simulink model "CL_MI_ARMAX"  (R2015a)
settings: Solver=ode45  StartTime=0.0  StopTime=520  RelTol=1e-3
values from neighbouring files (symbols this model uses):
  lambda = 1    [generar_prbs.m]    (also in parametros_ident.m = 0.995)
  Ts = 0.01    [generar_prbs.m]
libraries: dspsigops x2
settings Model: Creator=u_labelectro  LastModifiedBy=ARTURO
settings DataIOCC: SignalLoggingSaveFormat=ModelDataLogs
settings DebuggingCC: UnderspecifiedInitializationDetection=Classic  MergeDetectMultiDrivingBlocksExec=none  SolverPrmCheckMsg=warning  MultiTaskDSMMsg=warning  MultiTaskCondExecSysMsg=none  StateNameClashWarn=warning

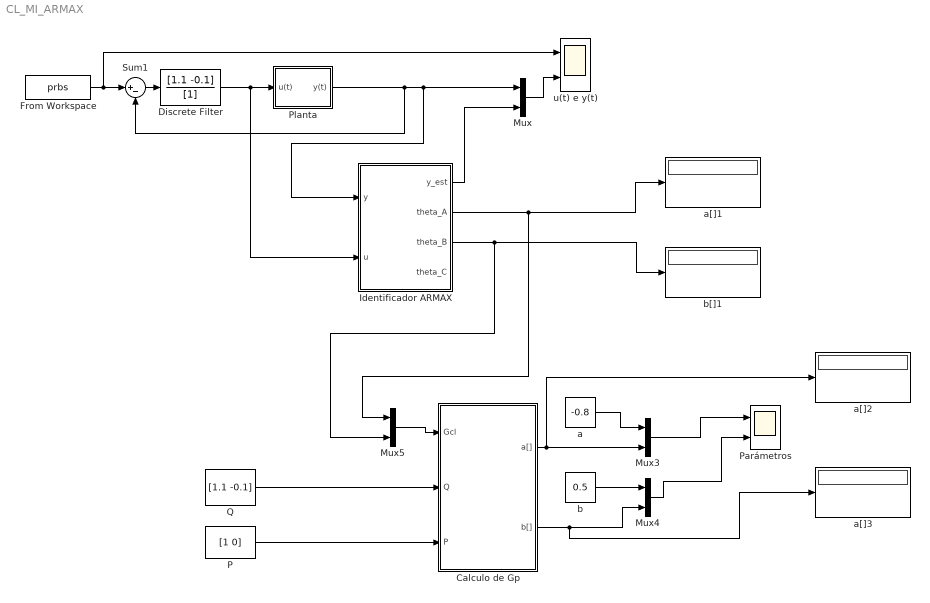
== system CL_MI_ARMAX ==
  Calculo de Gp : Subsystem
  Discrete Filter : DiscreteFilter  Numerator=[1.1 -0.1]  Denominator=[1]
  From Workspace : FromWorkspace  VariableName=prbs  SampleTime=Ts
  Identificador ARMAX : Subsystem
  Mux{,3..5} (4 alike) : Mux  Inputs=2
  P : Constant  Value=[1 0]
  Parámetros : Scope  NumInputPorts=2
      settings: YMin=-5~-5  YMax=5~5  SaveName=ScopeData4
  Planta : Subsystem
  Q : Constant  Value=[1.1 -0.1]
  Sum1 : Sum  Inputs=|+-
  a : Constant  Value=-0.8
  a[]1 : Display
  a[]2 : Display
  a[]3 : Display
  b : Constant  Value=0.5
  b[]1 : Display
  u(t) e y(t) : Scope  NumInputPorts=2
      settings: YMin=-5~-5  YMax=5~5
  wires:
  Identificador ARMAX/1(y_est) -> Mux/2
  Identificador ARMAX/3(theta_B) -> Mux5/2, b[]1/1
  Mux/1 -> u(t) e y(t)/2
  Discrete Filter/1 -> Identificador ARMAX/2(u), Planta/1(u(t))
  From Workspace/1 -> Sum1/1, u(t) e y(t)/1
  Planta/1(y(t)) -> Sum1/2, Identificador ARMAX/1(y), Mux/1
  a/1 -> Mux3/1
  b/1 -> Mux4/1
  Mux3/1 -> Parámetros/1
  Mux4/1 -> Parámetros/2
  Calculo de Gp/2(b[]) -> a[]3/1, Mux4/2
  Mux5/1 -> Calculo de Gp/1(Gcl)
  Q/1 -> Calculo de Gp/2(Q)
  P/1 -> Calculo de Gp/3(P)
  Identificador ARMAX/2(theta_A) -> Mux5/1, a[]1/1
  Calculo de Gp/1(a[]) -> a[]2/1, Mux3/2
  Sum1/1 -> Discrete Filter/1

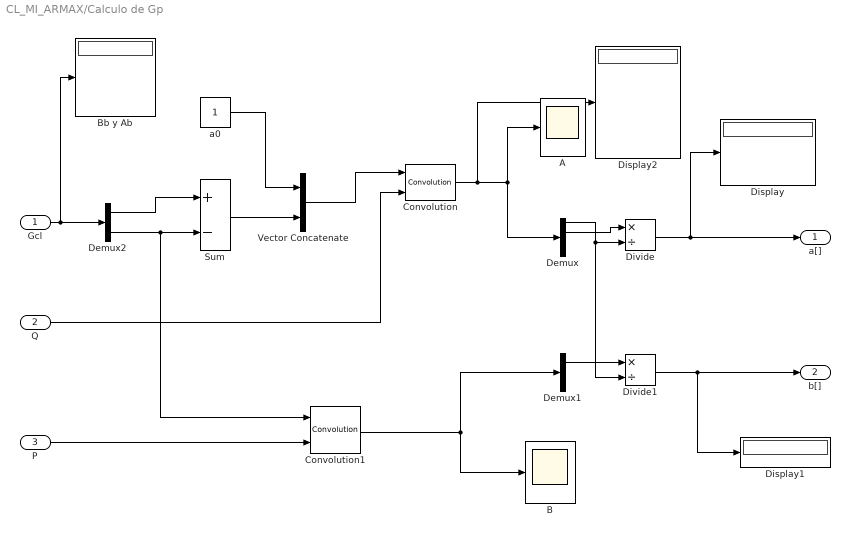
== system CL_MI_ARMAX/Calculo de Gp ==
  Gcl : Inport
  Q : Inport  Port=2
  P : Inport  Port=3
  A : Scope
      settings: SaveName=ScopeData2
  B : Scope
      settings: SaveName=ScopeData3
  "Bb y Ab " : Display
  Convolution : dspsigops/Convolution  domain=Time  outputDataTypeStr=Inherit: Same as accumulator  outputLastDataTypeStr=Inherit: Same as accumulator  outputMin=[]  outputMax=[]  roundingMode=Floor  overflowMode=off
  Convolution1 : dspsigops/Convolution  domain=Time  outputDataTypeStr=Inherit: Same as accumulator  outputLastDataTypeStr=Inherit: Same as accumulator  outputMin=[]  outputMax=[]  roundingMode=Floor  overflowMode=off
  Demux : Demux
  Demux1 : Demux  Outputs=3
  Demux2 : Demux  Outputs=2
  Display : Display
  Display1 : Display
  Display2 : Display
  Divide : Product  Inputs=*/
  Divide1 : Product  Inputs=*/
  Sum : Sum  Inputs=+-
  Vector Concatenate : Concatenate
  a0 : Constant
  a[] : Outport
  b[] : Outport  Port=2
  wires:
  Gcl/1 -> "Bb y Ab "/1, Demux2/1
  Demux2/2 -> Convolution1/1, Sum/2
  Demux2/1 -> Sum/1
  a0/1 -> Vector Concatenate/1
  Sum/1 -> Vector Concatenate/2
  Divide1/1 -> Display1/1, b[]/1
  Divide/1 -> Display/1, a[]/1
  Demux1/1 -> Divide1/1
  Demux/1 -> Divide/2, Divide1/2
  Demux/2 -> Divide/1
  Convolution1/1 -> Demux1/1, B/1
  Convolution/1 -> Display2/1, A/1, Demux/1
  Vector Concatenate/1 -> Convolution/1
  Q/1 -> Convolution/2
  P/1 -> Convolution1/2

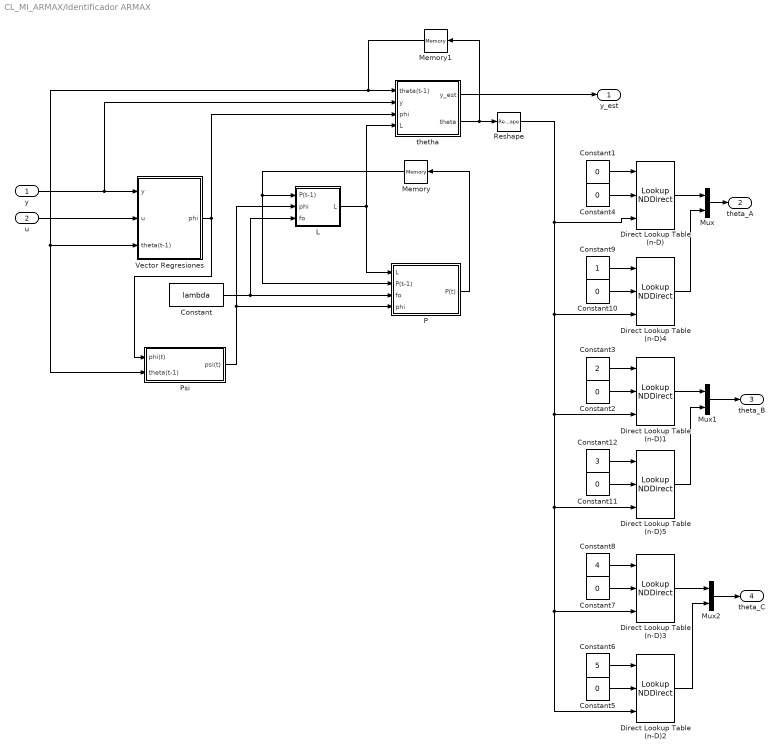
== system CL_MI_ARMAX/Identificador ARMAX ==
  y : Inport
  u : Inport  Port=2
  Constant : Constant  Value=lambda
  Constant{1..2,4..5,7,10..11} (7 alike) : Constant  Value=0
  Constant12 : Constant  Value=3
  Constant3 : Constant  Value=2
  Constant6 : Constant  Value=5
  Constant8 : Constant  Value=4
  Constant9 : Constant
  Direct Lookup Table (n-D){,1..5} (6 alike) : LookupNDDirect  TableIsInput=on
  L : Subsystem
  Memory : Memory  X0=1e6*eye(6)
  Memory1 : Memory
  Mux : Mux  Inputs=2
  Mux1 : Mux  Inputs=2
  Mux2 : Mux  Inputs=2
  P : Subsystem
  Psi : Subsystem
  Reshape : Reshape  OutputDimensionality=Column vector (2-D)
  Vector Regresiones : Subsystem
  thetha : Subsystem
  y_est : Outport
  theta_A : Outport  Port=2
  theta_B : Outport  Port=3
  theta_C : Outport  Port=4
  wires:
  y/1 -> thetha/2(y), Vector Regresiones/1(y)
  u/1 -> Vector Regresiones/2(u)
  L/1(L) -> thetha/4(L), P/1(L)
  P/1(P(t)) -> Memory/1
  Memory/1 -> P/2(P(t-1)), L/1(P(t-1))
  thetha/2(theta) -> Memory1/1, Reshape/1
  Memory1/1 -> Vector Regresiones/3(theta(t-1)), Psi/2(theta(t-1)), thetha/1(theta(t-1))
  thetha/1(y_est) -> y_est/1
  Constant1/1 -> Direct Lookup Table (n-D)/1
  Constant4/1 -> Direct Lookup Table (n-D)/2
  Constant3/1 -> Direct Lookup Table (n-D)1/1
  Constant2/1 -> Direct Lookup Table (n-D)1/2
  Constant/1 -> L/3(fo), P/3(fo)
  Psi/1(psi(t)) -> L/2(phi), P/4(phi)
  Vector Regresiones/1(phi) -> Psi/1(phi(t)), thetha/3(phi)
  Constant5/1 -> Direct Lookup Table (n-D)2/2
  Constant6/1 -> Direct Lookup Table (n-D)2/1
  Constant7/1 -> Direct Lookup Table (n-D)3/2
  Constant8/1 -> Direct Lookup Table (n-D)3/1
  Constant9/1 -> Direct Lookup Table (n-D)4/1
  Constant10/1 -> Direct Lookup Table (n-D)4/2
  Constant12/1 -> Direct Lookup Table (n-D)5/1
  Constant11/1 -> Direct Lookup Table (n-D)5/2
  Reshape/1 -> Direct Lookup Table (n-D)5/3, Direct Lookup Table (n-D)2/3, Direct Lookup Table (n-D)3/3, Direct Lookup Table (n-D)1/3, Direct Lookup Table (n-D)4/3, Direct Lookup Table (n-D)/3
  Direct Lookup Table (n-D)/1 -> Mux/1
  Mux/1 -> theta_A/1
  Direct Lookup Table (n-D)4/1 -> Mux/2
  Mux2/1 -> theta_C/1
  Mux1/1 -> theta_B/1
  Direct Lookup Table (n-D)1/1 -> Mux1/1
  Direct Lookup Table (n-D)5/1 -> Mux1/2
  Direct Lookup Table (n-D)3/1 -> Mux2/1
  Direct Lookup Table (n-D)2/1 -> Mux2/2

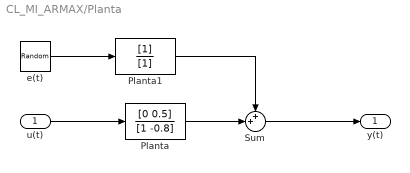
== system CL_MI_ARMAX/Planta ==
  u(t) : Inport
  Planta : DiscreteFilter  Numerator=[0 0.5]  Denominator=[1 -0.8]  SampleTime=Ts
  Planta1 : DiscreteFilter  Denominator=[1]  SampleTime=Ts
  Sum : Sum  Inputs=++|
  e(t) : RandomNumber  Variance=0.0001  SampleTime=Ts
  y(t) : Outport
  wires:
  e(t)/1 -> Planta1/1
  Planta1/1 -> Sum/1
  Planta/1 -> Sum/2
  u(t)/1 -> Planta/1
  Sum/1 -> y(t)/1

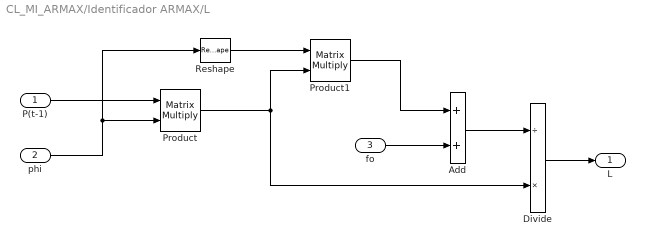
== system CL_MI_ARMAX/Identificador ARMAX/L ==
  P(t-1) : Inport
  phi : Inport  Port=2
  fo : Inport  Port=3
  Add : Sum
  Divide : Product  Inputs=/*
  Product : Product  Multiplication=Matrix(*)
  Product1 : Product  Multiplication=Matrix(*)
  Reshape : Reshape  OutputDimensionality=Row vector (2-D)
  L : Outport
  wires:
  phi/1 -> Reshape/1, Product/2
  P(t-1)/1 -> Product/1
  Reshape/1 -> Product1/1
  fo/1 -> Add/2
  Product1/1 -> Add/1
  Divide/1 -> L/1
  Add/1 -> Divide/1
  Product/1 -> Divide/2, Product1/2

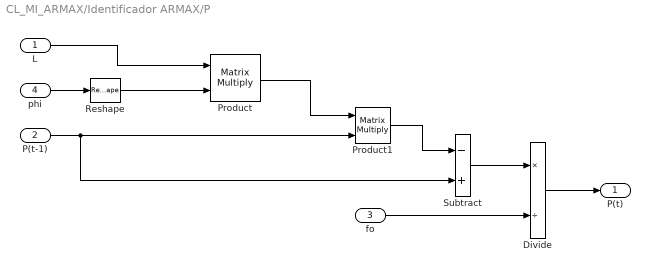
== system CL_MI_ARMAX/Identificador ARMAX/P ==
  L : Inport
  P(t-1) : Inport  Port=2
  fo : Inport  Port=3
  phi : Inport  Port=4
  Divide : Product  Inputs=*/
  Product : Product  Multiplication=Matrix(*)
  Product1 : Product  Multiplication=Matrix(*)
  Reshape : Reshape  OutputDimensionality=Row vector (2-D)
  Subtract : Sum  Inputs=-+
  P(t) : Outport
  wires:
  phi/1 -> Reshape/1
  Reshape/1 -> Product/2
  L/1 -> Product/1
  Product/1 -> Product1/1
  P(t-1)/1 -> Subtract/2, Product1/2
  Product1/1 -> Subtract/1
  Subtract/1 -> Divide/1
  fo/1 -> Divide/2
  Divide/1 -> P(t)/1

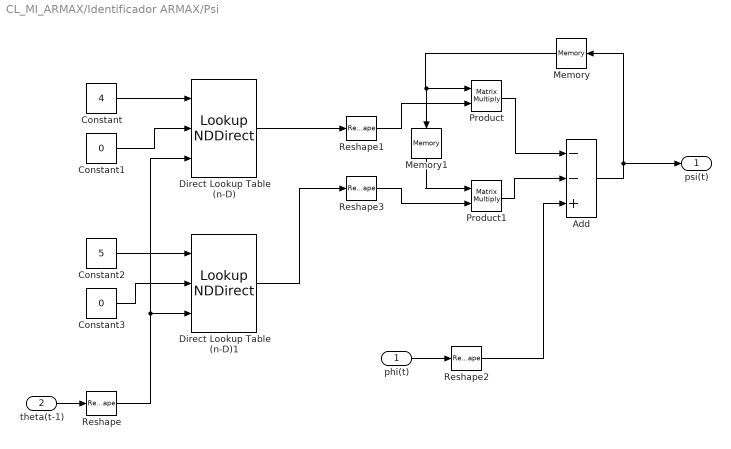
== system CL_MI_ARMAX/Identificador ARMAX/Psi ==
  phi(t) : Inport
  theta(t-1) : Inport  Port=2
  Add : Sum  Inputs=--+
  Constant : Constant  Value=4
  Constant1 : Constant  Value=0
  Constant2 : Constant  Value=5
  Constant3 : Constant  Value=0
  Direct Lookup Table (n-D) : LookupNDDirect  TableIsInput=on
  Direct Lookup Table (n-D)1 : LookupNDDirect  TableIsInput=on
  Memory : Memory
  Memory1 : Memory
  Product : Product  Multiplication=Matrix(*)
  Product1 : Product  Multiplication=Matrix(*)
  Reshape : Reshape  OutputDimensionality=Column vector (2-D)
  Reshape1 : Reshape  OutputDimensionality=Row vector (2-D)
  Reshape2 : Reshape  OutputDimensionality=Column vector (2-D)
  Reshape3 : Reshape  OutputDimensionality=Row vector (2-D)
  psi(t) : Outport
  wires:
  Constant/1 -> Direct Lookup Table (n-D)/1
  Constant1/1 -> Direct Lookup Table (n-D)/2
  theta(t-1)/1 -> Reshape/1
  Reshape/1 -> Direct Lookup Table (n-D)1/3, Direct Lookup Table (n-D)/3
  Reshape1/1 -> Product/2
  Product/1 -> Add/1
  phi(t)/1 -> Reshape2/1
  Add/1 -> Memory/1, psi(t)/1
  Constant2/1 -> Direct Lookup Table (n-D)1/1
  Constant3/1 -> Direct Lookup Table (n-D)1/2
  Direct Lookup Table (n-D)1/1 -> Reshape3/1
  Direct Lookup Table (n-D)/1 -> Reshape1/1
  Memory/1 -> Memory1/1, Product/1
  Reshape2/1 -> Add/3
  Product1/1 -> Add/2
  Reshape3/1 -> Product1/2
  Memory1/1 -> Product1/1

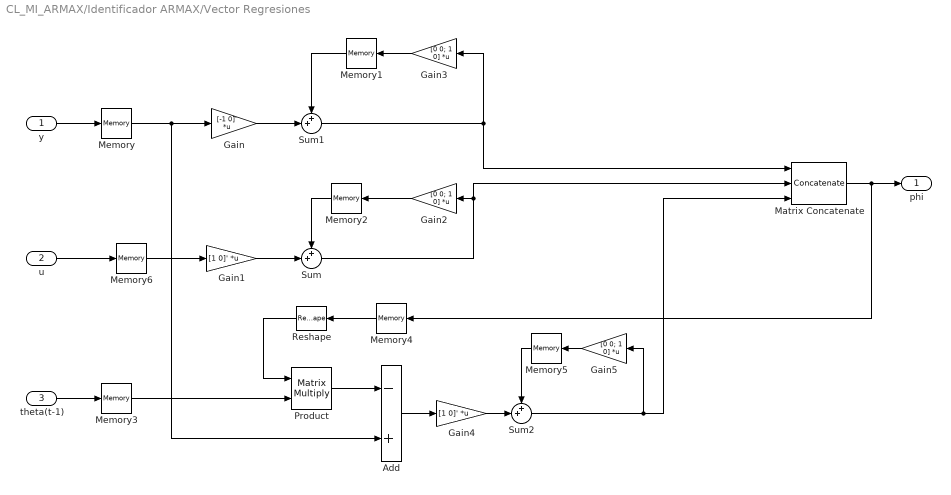
== system CL_MI_ARMAX/Identificador ARMAX/Vector Regresiones ==
  y : Inport
  u : Inport  Port=2
  theta(t-1) : Inport  Port=3
  Add : Sum  Inputs=-+
  Gain : Gain  Gain=[-1 0]'  Multiplication=Matrix(K*u)
  Gain1 : Gain  Gain=[1 0]'  Multiplication=Matrix(K*u)
  Gain2 : Gain  Gain=[0 0; 1 0]  Multiplication=Matrix(K*u)
  Gain3 : Gain  Gain=[0 0; 1 0]  Multiplication=Matrix(K*u)
  Gain4 : Gain  Gain=[1 0]'  Multiplication=Matrix(K*u)
  Gain5 : Gain  Gain=[0 0; 1 0]  Multiplication=Matrix(K*u)
  Matrix Concatenate : Concatenate  NumInputs=3  Mode=Multidimensional array
  Memory{,1..6} (7 alike) : Memory
  Product : Product  Multiplication=Matrix(*)
  Reshape : Reshape  OutputDimensionality=Row vector (2-D)
  Sum : Sum  Inputs=++|
  Sum1 : Sum  Inputs=++|
  Sum2 : Sum  Inputs=++|
  phi : Outport
  wires:
  y/1 -> Memory/1
  Memory2/1 -> Sum/1
  Gain1/1 -> Sum/2
  Gain2/1 -> Memory2/1
  Memory1/1 -> Sum1/1
  Gain3/1 -> Memory1/1
  Memory/1 -> Add/2, Gain/1
  Matrix Concatenate/1 -> Memory4/1, phi/1
  Sum1/1 -> Matrix Concatenate/1, Gain3/1
  Sum/1 -> Matrix Concatenate/2, Gain2/1
  theta(t-1)/1 -> Memory3/1
  Memory3/1 -> Product/2
  Reshape/1 -> Product/1
  Memory4/1 -> Reshape/1
  Product/1 -> Add/1
  Add/1 -> Gain4/1
  Gain4/1 -> Sum2/2
  Gain5/1 -> Memory5/1
  Memory5/1 -> Sum2/1
  Sum2/1 -> Gain5/1, Matrix Concatenate/3
  Gain/1 -> Sum1/2
  u/1 -> Memory6/1
  Memory6/1 -> Gain1/1

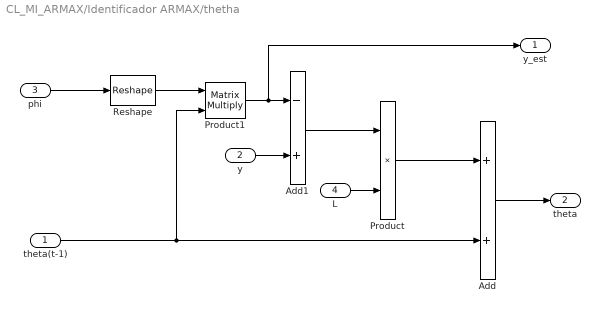
== system CL_MI_ARMAX/Identificador ARMAX/thetha ==
  theta(t-1) : Inport
  y : Inport  Port=2
  phi : Inport  Port=3
  L : Inport  Port=4
  Add : Sum
  Add1 : Sum  Inputs=-+
  Product : Product
  Product1 : Product  Multiplication=Matrix(*)
  Reshape : Reshape  OutputDimensionality=Row vector (2-D)
  y_est : Outport
  theta : Outport  Port=2
  wires:
  phi/1 -> Reshape/1
  y/1 -> Add1/2
  L/1 -> Product/2
  Add1/1 -> Product/1
  Product/1 -> Add/1
  theta(t-1)/1 -> Add/2, Product1/2
  Reshape/1 -> Product1/1
  Product1/1 -> y_est/1, Add1/1
  Add/1 -> theta/1
